simulink model "Q2_partf"  (R2018a)
settings: Solver=FixedStepDiscrete  StartTime=0  StopTime=0.10  RelTol=1e-3
libraries: powerlib x12, powerlib_meascontrol x3
settings Model: Creator=burya  LastModifiedBy=burya

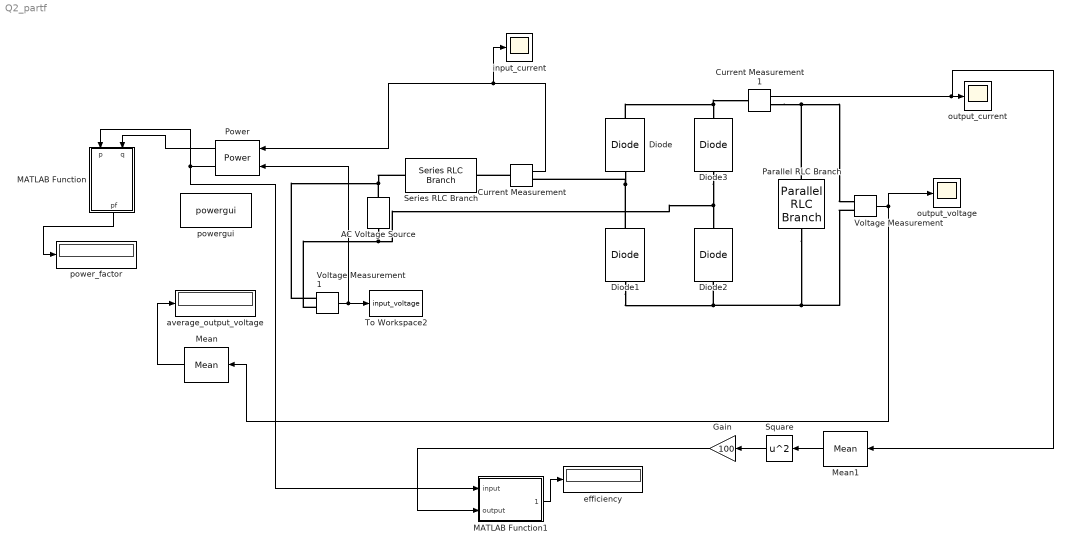
== system Q2_partf ==
  AC Voltage Source : powerlib/Electrical Sources/AC Voltage Source  Amplitude=230*sqrt(2)  Phase=0  Frequency=50  SampleTime=1e-6  Measurements=None  BusType=swing  Pref=10e3  Qref=0  Qmin=-inf  Qmax=+inf
  Current Measurement : powerlib/Measurements/Current Measurement  PhasorSimulation=off  OutputType=Complex  PSBequivalent=0
  Current Measurement1 : powerlib/Measurements/Current Measurement  PhasorSimulation=off  OutputType=Complex  PSBequivalent=0
  Diode{,1..3} (4 alike) : powerlib/Power Electronics/Diode  Ron=1e-9  Lon=0  Vf=1.1  IC=0  UseSnubber=0  Rs=500  Cs=300e-12  Measurements=off
  Gain : Gain  Gain=100
  MATLAB Function : MATLAB Function  TreatAsAtomicUnit=on
  MATLAB Function1 : MATLAB Function  TreatAsAtomicUnit=on
  Mean : powerlib_meascontrol/Measurements/Mean  Freq=50  Vinit=0  Ts=1e-6
  Mean1 : powerlib_meascontrol/Measurements/Mean  Freq=50  Vinit=0  Ts=1e-6
  Parallel RLC Branch : powerlib/Elements/Parallel RLC Branch  LConnTagsString=a  RConnTagsString=__new0  BranchType=RC  Resistance=100  Inductance=1e-3  SetiL0=off  InitialCurrent=0  Capacitance=2.5e-3  Setx0=on  InitialVoltage=230*sqrt(2)  Measurements=None
  Power : powerlib_meascontrol/Measurements/Power  Freq=50  Vinit=[1, 0]  Iinit=[1, 0]  Ts=1e-6
      settings: SourceProductName=Simscape Power Systems
  Series RLC Branch : powerlib/Elements/Series RLC Branch  LConnTagsString=__new0  RConnTagsString=__new0  BranchType=RL  Resistance=1e-3  Inductance=1e-3  SetiL0=off  InitialCurrent=0  Capacitance=1e-6  Setx0=off  InitialVoltage=0  Measurements=None
  Square : Math  Operator=square  SaturateOnIntegerOverflow=on
  To Workspace2 : ToWorkspace  VariableName=input_voltage  SaveFormat=Structure With Time  SampleTime=-1
  Voltage Measurement : powerlib/Measurements/Voltage Measurement  PhasorSimulation=off  OutputType=Complex  PSBequivalent=0
  Voltage Measurement1 : powerlib/Measurements/Voltage Measurement  PhasorSimulation=off  OutputType=Complex  PSBequivalent=0
  average_output_voltage : Display
  efficiency : Display
  input_current : Scope
  "output_current " : Scope
  output_voltage : Scope
  "power_factor " : Display
  powergui : powerlib/powergui  Priority=1  SimulationMode=Discrete  SampleTime=1e-6  frequency=60  Iterations=50  frequencyindice=50  Pbase=100e6  ErrMax=1e-4  UnitsV=kV  UnitsW=MW  buscounter=0  FunctionMessages=off  echomessages=off  EnableUseOfTLC=off  CurrentSourceSwitches=off  DisableSnubberDevices=off  DisableRonSwitches=off  DisableVfSwitches=off  DisplayEquations=off  SolverType=Tustin/Backward Euler (TBE)  Interpol=off  ExternalGateDelay=off  methode=off  Ts=100  x0status=blocks  SPID=off  SwTol=0  HookPort=off  RestoreLinks=warning  ResistiveCurrentMeasurement=off  Frange=[0:2:500]  Ylog=off  Xlog=on  ShowGrid=off  save=off  variable=ZData  structure=input_current  ZoomFFT=off  StartTime=0.02  cycles=1  DisplayStyle=1  fundamental=50  FreqAxis=off  MaxFrequency=950  frequencyindicesteady=1  RmsSteady=1  display=off
  wires:
  Current Measurement/1 -> input_current/1, Power/2
  Voltage Measurement/1 -> output_voltage/1, Mean/1
  Voltage Measurement1/1 -> Power/1, To Workspace2/1
  Mean/1 -> average_output_voltage/1
  Power/1 -> MATLAB Function1/1(input), MATLAB Function/1(p)
  Power/2 -> MATLAB Function/2(q)
  MATLAB Function/1(pf) -> "power_factor "/1
  Current Measurement1/1 -> "output_current "/1, Mean1/1
  MATLAB Function1/1(efficiency) -> efficiency/1
  Mean1/1 -> Square/1
  Gain/1 -> MATLAB Function1/2(output)
  Square/1 -> Gain/1
  connections:
  AC Voltage Source/RConn1 -- Series RLC Branch/LConn1 -- Voltage Measurement1/LConn1
  Diode3/LConn1 -- Voltage Measurement1/LConn2 -- AC Voltage Source/LConn1 -- Diode2/RConn1
  Diode1/RConn1 -- Diode/LConn1 -- Current Measurement/RConn1
  Diode1/LConn1 -- Voltage Measurement/LConn2 -- Parallel RLC Branch/RConn1 -- Diode2/LConn1
  Parallel RLC Branch/LConn1 -- Current Measurement1/RConn1 -- Voltage Measurement/LConn1
  Current Measurement/LConn1 -- Series RLC Branch/RConn1
  Diode/RConn1 -- Current Measurement1/LConn1 -- Diode3/RConn1

== matlab function Q2_partf/MATLAB Function1 ==
  data: input input; efficiency output; output input
function efficiency = fcn(input,output)

efficiency = (output/input)*100;

== matlab function Q2_partf/MATLAB Function ==
  data: p input; pf output; q input
function pf = fcn(p,q)

pf=p/sqrt(p^2+q^2);
